simulink library "surfaceCoefficients_ul"  (R2018b)
settings: Solver=VariableStepAuto  StartTime=0.0  StopTime=10.0  RelTol=1e-3
undefined symbols (not defined in the file): aeroStruct, vhcl
libraries: dspstat3 x2, dsppolyfun x2
settings Model: Creator=mcobb  LastModifiedBy=Josh Gaming

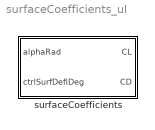
== system surfaceCoefficients_ul ==
  surfaceCoefficients : Subsystem

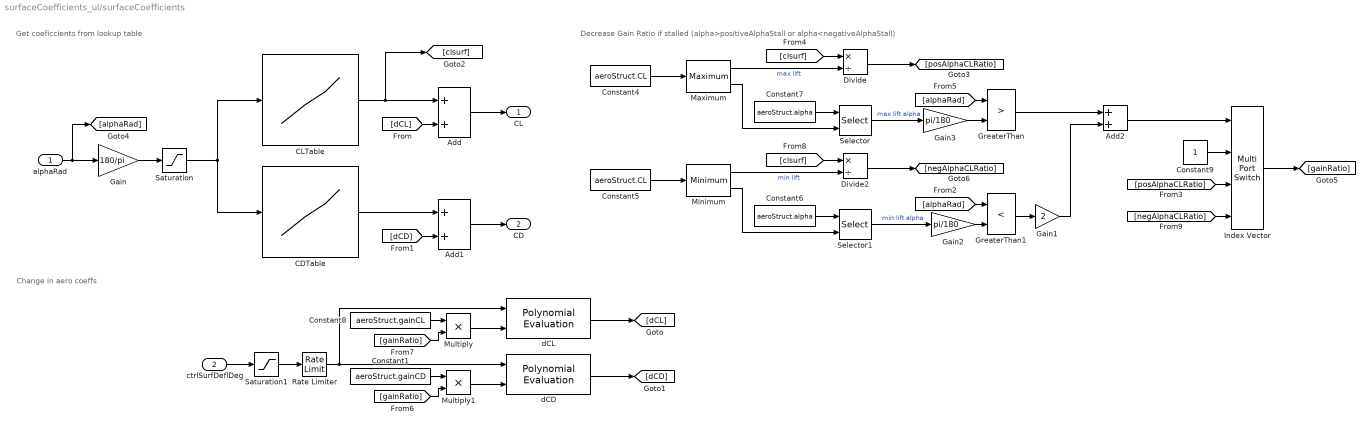
== system surfaceCoefficients_ul/surfaceCoefficients ==
  note: Get coeficcients from lookup table
  note: Decrease Gain Ratio if stalled (alpha>positiveAlphaStall or alpha<negativeAlphaStall)
  note: Change in aero coeffs
  alphaRad : Inport
  ctrlSurfDeflDeg : Inport  Port=2
  Add : Sum
  Add1 : Sum
  Add2 : Sum
  CDTable : Lookup_n-D  NumberOfTableDimensions=1  LookupTableObject=CLTable  BreakpointsForDimension1=aeroStruct.alpha  Table=aeroStruct.CD  ExtrapMethod=Clip  UseLastTableValue=on  InternalRulePriority=Speed  RndMeth=Simplest  InputSameDT=on
  CLTable : Lookup_n-D  NumberOfTableDimensions=1  LookupTableObject=CLTable  BreakpointsForDimension1=aeroStruct.alpha  Table=aeroStruct.CL  ExtrapMethod=Clip  UseLastTableValue=on  InternalRulePriority=Speed  RndMeth=Simplest  InputSameDT=on
  Constant1 : Constant  Value=aeroStruct.gainCD
  Constant4 : Constant  Value=aeroStruct.CL
  Constant5 : Constant  Value=aeroStruct.CL
  Constant6 : Constant  Value=aeroStruct.alpha
  Constant7 : Constant  Value=aeroStruct.alpha
  Constant8 : Constant  Value=aeroStruct.gainCL
  Constant9 : Constant
  Divide : Product  Inputs=*/
  Divide2 : Product  Inputs=*/
  Gain : Gain  Gain=180/pi
  Gain1 : Gain  Gain=2
  Gain2 : Gain  Gain=pi/180
  Gain3 : Gain  Gain=pi/180
  GreaterThan : RelationalOperator  Operator=>  OutDataTypeStr=boolean  RndMeth=Simplest
  GreaterThan1 : RelationalOperator  Operator=<  OutDataTypeStr=boolean  RndMeth=Simplest
  Index Vector : MultiPortSwitch  DataPortOrder=Zero-based contiguous  zeroidx=on
  Maximum : dspstat3/Maximum  operation=maximum  fcn=Value and Index  indexBase=One  operateOver=Each column  Dimension=1  InputProcessing=Columns as channels (frame based)  reset=None  roiEnable=off  roiType=Rectangles  roiPortion=Entire ROI  roiOutput=Individual statistics for each ROI  roiFlag=off  roundingMode=Floor  overflowMode=off  accumDataTypeStr=Inherit: Same as product output  accumLastDataTypeStr=Inherit: Same as product output
  Minimum : dspstat3/Minimum  operation=minimum  fcn=Value and Index  indexBase=One  operateOver=Each column  Dimension=1  InputProcessing=Columns as channels (frame based)  reset=None  roiEnable=off  roiType=Rectangles  roiPortion=Entire ROI  roiOutput=Individual statistics for each ROI  roiFlag=off  roundingMode=Floor  overflowMode=off
      settings: SourceProductName=DSP System Toolbox  SourceProductBaseCode=DS
  Multiply : Product
  Multiply1 : Product
  Rate Limiter : RateLimiter  RisingSlewLimit=aeroStruct.maxCtrlDefSpeed  FallingSlewLimit=-aeroStruct.maxCtrlDefSpeed  SampleTimeMode=inherited
  Saturation : Saturate  UpperLimit=90  LowerLimit=-90
  Saturation1 : Saturate  UpperLimit=aeroStruct.maxCtrlDef  LowerLimit=aeroStruct.minCtrlDef
  Selector : Selector  InputPortWidth=length(vhcl.portWing.alpha.Value)  IndexOptions=Index vector (port)  Indices=[1 3]  OutputSizes=1
  Selector1 : Selector  InputPortWidth=length(vhcl.portWing.alpha.Value)  IndexOptions=Index vector (port)  Indices=[1 3]  OutputSizes=1
  dCD : dsppolyfun/Polynomial Evaluation  useConstCoeffs=off  constCoeffs=[0]
      settings: SourceProductName=DSP System Toolbox  SourceProductBaseCode=DS
  dCL : dsppolyfun/Polynomial Evaluation  useConstCoeffs=off  constCoeffs=[0]
      settings: SourceProductName=DSP System Toolbox  SourceProductBaseCode=DS
  CL : Outport
  CD : Outport  Port=2
  wires:
  Gain/1 -> Saturation/1
  dCL/1 -> [dCL]
  dCD/1 -> [dCD]
  [dCL] -> Add/2
  CLTable/1 -> [clsurf], Add/1
  Add/1 -> CL/1
  Add1/1 -> CD/1
  [dCD] -> Add1/2
  CDTable/1 -> Add1/1
  Multiply1/1 -> dCD/2
  Rate Limiter/1 -> dCL/1, dCD/1
  ctrlSurfDeflDeg/1 -> Saturation1/1
  Saturation/1 -> CLTable/1, CDTable/1
  Constant4/1 -> Maximum/1
  alphaRad/1 -> [alphaRad], Gain/1
  Constant7/1 -> Selector/1
  Maximum/2 -> Selector/2
  Selector/1 -> Gain3/1  "max lift alpha"
  Divide/1 -> [posAlphaCLRatio]
  Maximum/1 -> Divide/2  "max lift"
  [clsurf] -> Divide/1
  [alphaRad] -> GreaterThan/1
  Minimum/2 -> Selector1/2
  [clsurf] -> Divide2/1
  Divide2/1 -> [negAlphaCLRatio]
  Minimum/1 -> Divide2/2  "min lift"
  Constant6/1 -> Selector1/1
  Constant5/1 -> Minimum/1
  Selector1/1 -> Gain2/1  "min lift alpha"
  [alphaRad] -> GreaterThan1/1
  GreaterThan1/1 -> Gain1/1
  GreaterThan/1 -> Add2/1
  Gain1/1 -> Add2/2
  Add2/1 -> Index Vector/1
  Constant9/1 -> Index Vector/2
  [negAlphaCLRatio] -> Index Vector/4
  [posAlphaCLRatio] -> Index Vector/3
  Index Vector/1 -> [gainRatio]
  Constant8/1 -> Multiply/1
  [gainRatio] -> Multiply/2
  Multiply/1 -> dCL/2
  [gainRatio] -> Multiply1/2
  Constant1/1 -> Multiply1/1
  Gain2/1 -> GreaterThan1/2
  Gain3/1 -> GreaterThan/2
  Saturation1/1 -> Rate Limiter/1
